simulink model "FlSys_CalcCnvFac"  (R2016b)
settings: configuration reference "CodeGenConfigSet" (kept outside this file)
values from neighbouring files (symbols this model uses):
  FlSys_facStoich_C = Calibration.Parameter    [init_FlSys_CalcCnvFac.m]
  FlSys_rhoFl_C = Calibration.Parameter    [init_FlSys_CalcCnvFac.m]
  FlSys_rhoFl_CUR = Calibration.Parameter    [init_FlSys_CalcCnvFac.m]
  FlSys_rhoFl_CURX = Calibration.Parameter    [init_FlSys_CalcCnvFac.m]
  FlSys_rhoFlCnvFac_C = Calibration.Parameter    [init_FlSys_CalcCnvFac.m]
  FlSys_swtRhoFlCnv_C = Calibration.Parameter    [init_FlSys_CalcCnvFac.m]
settings Model: Creator=Administrator  LastModifiedBy=wangrui
settings ConfigSetRef: SourceLocation=Base Workspace

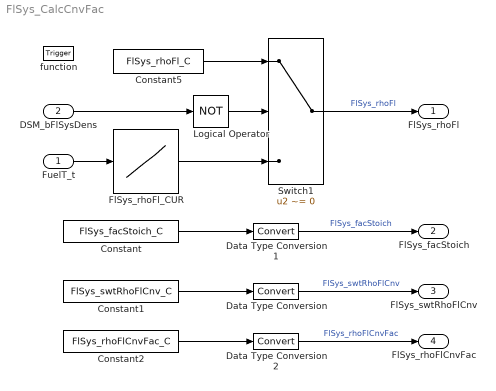
== system FlSys_CalcCnvFac ==
  FuelT_t : Inport  Tag=deg  Description=Temperature of fuel  OutMin=-50  OutMax=150  OutDataTypeStr=Temp_deg
  DSM_bFlSysDens : Inport  Description=Status of FId_FlSysDens  Port=2  OutMin=0  OutMax=1  OutDataTypeStr=boolean
  function : TriggerPort  TriggerType=function-call  VariantControl=Variant
  Constant : Constant  Value=FlSys_facStoich_C
  Constant1 : Constant  Value=FlSys_swtRhoFlCnv_C
  Constant2 : Constant  Value=FlSys_rhoFlCnvFac_C
  Constant5 : Constant  Value=FlSys_rhoFl_C
  Data Type Conversion : DataTypeConversion
  Data Type Conversion1 : DataTypeConversion
  Data Type Conversion2 : DataTypeConversion
  FlSys_rhoFl_CUR : Lookup_n-D  NumberOfTableDimensions=1  BreakpointsForDimension1=FlSys_rhoFl_CURX  IndexSearchMethod=Linear search  BeginIndexSearchUsingPreviousIndexResult=on  Table=FlSys_rhoFl_CUR  ExtrapMethod=Clip  UseLastTableValue=on  InternalRulePriority=Speed  OutDataTypeStr=Inherit: Inherit via back propagation  SaturateOnIntegerOverflow=on
  Logical Operator : Logic  Operator=NOT  AllPortsSameDT=off  OutDataTypeStr=boolean
  Switch1 : Switch  Criteria=u2 ~= 0  SaturateOnIntegerOverflow=on  InputSameDT=on
  FlSys_rhoFl : Outport  Tag=kg/m^3  Description=Fuel density coefficient  OutMin=0  OutMax=3276  OutDataTypeStr=Fuel_Rho_kg_m3
  FlSys_facStoich : Outport  Description=Stochiometric fuel factor  Port=2  OutMin=-32  OutMax=31  OutDataTypeStr=Factor
  FlSys_swtRhoFlCnv : Outport  Description=switch for customer specific fuel conversion factor  Port=3  OutDataTypeStr=Enum: Switch_conv
  FlSys_rhoFlCnvFac : Outport  Tag=kg/m^3  Description=customer specific fuel conversion factor  Port=4  OutMin=0  OutMax=3276  OutDataTypeStr=Fuel_Rho_kg_m3
  wires:
  FuelT_t/1 -> FlSys_rhoFl_CUR/1
  Constant5/1 -> Switch1/1
  DSM_bFlSysDens/1 -> Logical Operator/1
  FlSys_rhoFl_CUR/1 -> Switch1/3
  Switch1/1 -> FlSys_rhoFl/1  "FlSys_rhoFl"
  Logical Operator/1 -> Switch1/2
  Constant/1 -> Data Type Conversion1/1
  Constant1/1 -> Data Type Conversion/1
  Constant2/1 -> Data Type Conversion2/1
  Data Type Conversion1/1 -> FlSys_facStoich/1  "FlSys_facStoich"
  Data Type Conversion/1 -> FlSys_swtRhoFlCnv/1  "FlSys_swtRhoFlCnv"
  Data Type Conversion2/1 -> FlSys_rhoFlCnvFac/1  "FlSys_rhoFlCnvFac"
